simulink model "selector_port_test"  (Simulink 8.4)
settings: Solver=VariableStepDiscrete  StartTime=0.0  StopTime=0  MaxStep=1  RelTol=1e-3
settings Model: Creator=arnaud  LastModifiedBy=arnaud
settings DataIOCC: ExternalInput=xin  SaveFormat=Structure

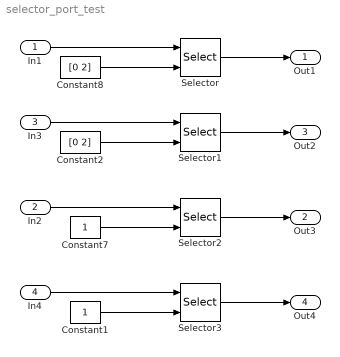
== system selector_port_test ==
  In1 : Inport  PortDimensions=3
  In2 : Inport  Port=2  PortDimensions=3
  In3 : Inport  Port=3  PortDimensions=3
  In4 : Inport  Port=4  PortDimensions=3
  Constant1 : Constant
  Constant2 : Constant  Value=[0 2]
  Constant7 : Constant
  Constant8 : Constant  Value=[0 2]
  Selector : Selector  IndexMode=Zero-based  InputPortWidth=3  IndexOptions=Index vector (port)  Indices=[1 0 0]
  Selector1 : Selector  IndexMode=Zero-based  InputPortWidth=3  IndexOptions=Index vector (port)  Indices=[1 0 0]
  Selector2 : Selector  InputPortWidth=3  IndexOptions=Index vector (port)  Indices=2
  Selector3 : Selector  IndexMode=Zero-based  InputPortWidth=3  IndexOptions=Index vector (port)  Indices=2  OutputSizes=2
  Out1 : Outport
  Out3 : Outport  Port=2
  Out2 : Outport  Port=3
  Out4 : Outport  Port=4
  wires:
  Selector/1 -> Out1/1
  In1/1 -> Selector/1
  Selector2/1 -> Out3/1
  In2/1 -> Selector2/1
  Constant8/1 -> Selector/2
  Constant7/1 -> Selector2/2
  Selector1/1 -> Out2/1
  In3/1 -> Selector1/1
  Selector3/1 -> Out4/1
  In4/1 -> Selector3/1
  Constant2/1 -> Selector1/2
  Constant1/1 -> Selector3/2
